simulink model "State_Space_model"  (R2018a)
settings: Solver=ode45  StartTime=0.0  StopTime=5  RelTol=1e-3  EnableMultiTasking=on
values from neighbouring files (symbols this model uses):
  A = [0 0 0   0    0  0     0 ... (first row only)    [State_Space_Pneumatic_Damper.m]
  am1 = 2*zetta*Wn    (= 11.2)    [State_Space_Pneumatic_Damper.m]
  am2 = Wn^2    (= 64)    [State_Space_Pneumatic_Damper.m]
  B = [   c3 ... (first row only)    [State_Space_Pneumatic_Damper.m]
  bm = am2    (= 64)    [State_Space_Pneumatic_Damper.m]
  C = [1 0 0 0 0 0 0 ... (first row only)    [State_Space_Pneumatic_Damper.m]
  D = [0 ... (first row only)    [State_Space_Pneumatic_Damper.m]
  h0 = 150    [State_Space_Pneumatic_Damper.m]
settings Model: Creator=ahmad  LastModifiedBy=Ahmad
settings DataIOCC: LimitDataPoints=on  SaveFormat=Array
settings OptimizationCC: LifeSpan=inf
settings DebuggingCC: UnderspecifiedInitializationDetection=Classic  MergeDetectMultiDrivingBlocksExec=none  SolverPrmCheckMsg=warning  StateNameClashWarn=warning  SFUnexpectedBacktrackingDiag=warning  SFNoUnconditionalDefaultTransitionDiag=warning  SFExecutionAtInitializationDiag=none
settings HardwareCC: ProdBitPerPointer=32  ProdBitPerSizeT=32  ProdBitPerPtrDiffT=32  ProdLargestAtomicFloat=None  ProdIntDivRoundTo=Undefined  ProdEndianess=Unspecified  ProdWordSize=32  ProdHWDeviceType=32-bit Generic
settings ModelReferenceCC: PropagateSignalLabelsOutOfModel=off
settings CodeAppCC: StateflowObjectComments=on
settings GRTTargetCC: TargetLangStandard=C89/C90 (ANSI)  GeneratePreprocessorConditionals=Disable all
settings ConfigComp: CovMetricSettings=dw  CovHtmlReporting=on  CovSaveCumulativeToWorkspaceVar=on  CovSaveSingleToWorkspaceVar=on  CovExternalEMLEnable=off

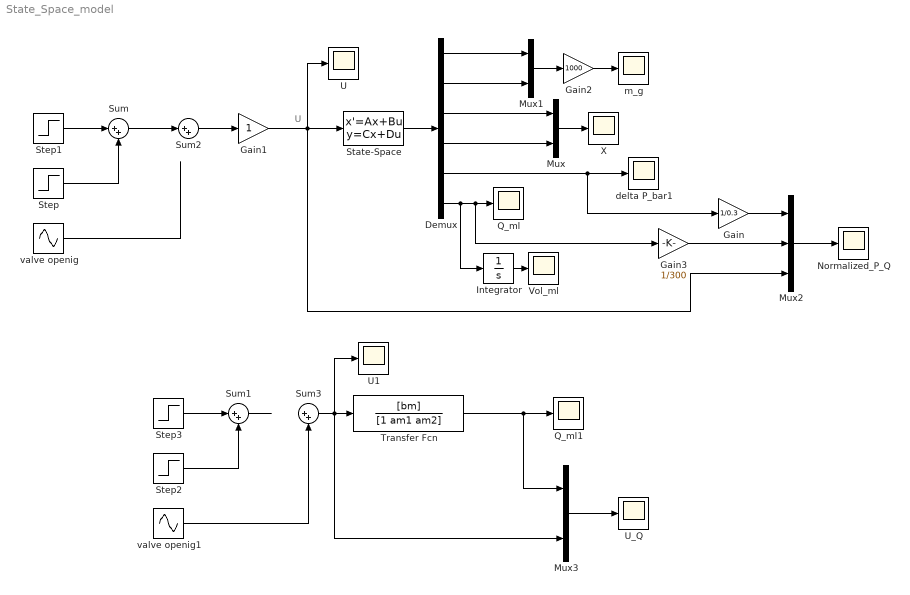
== system State_Space_model ==
  note: U
  Demux : Demux  Outputs=6
  Gain : Gain  Gain=1/0.3
  Gain1 : Gain
  Gain2 : Gain  Gain=1000
  Gain3 : Gain  Gain=1/300
  Integrator : Integrator
  Mux : Mux  Inputs=2
  Mux1 : Mux  Inputs=2
  Mux2 : Mux  Inputs=3
  Mux3 : Mux  Inputs=2
  Normalized_P_Q : Scope
  Q_ml : Scope
  Q_ml1 : Scope
  State-Space : StateSpace  A=A  B=B  C=C  D=D  InitialCondition=[0 0 1.5 1.5 h0/2 h0/2 0]
  Step : Step  Time=0.1  After=-1  SampleTime=0
  Step1 : Step  Time=0  SampleTime=0
  Step2 : Step  Time=0.1  After=-1  SampleTime=0
  Step3 : Step  Time=0  SampleTime=0
  Sum{,1..3} (4 alike) : Sum  Inputs=|++
  Transfer Fcn : TransferFcn  Numerator=[bm]  Denominator=[1 am1 am2]
  U : Scope
  U1 : Scope
  U_Q : Scope
  Vol_ml : Scope
  X : Scope
  delta P_bar1 : Scope
  m_g : Scope
  valve openig : Sin  Phase=pi/2  SampleTime=0
  valve openig1 : Sin  Frequency=8.3  SampleTime=0
  wires:
  State-Space/1 -> Demux/1
  valve openig/1 -> ?
  Demux/6 -> Gain3/1, Q_ml/1, Integrator/1
  Sum/1 -> Sum2/1
  Step/1 -> Sum/2
  Step1/1 -> Sum/1
  Integrator/1 -> Vol_ml/1
  Sum2/1 -> Gain1/1
  Demux/1 -> Mux1/1
  Demux/3 -> Mux/1
  Demux/4 -> Mux/2
  Gain2/1 -> m_g/1
  Demux/2 -> Mux1/2
  Mux/1 -> X/1
  Mux1/1 -> Gain2/1
  Demux/5 -> Gain/1, delta P_bar1/1
  Mux2/1 -> Normalized_P_Q/1
  Gain/1 -> Mux2/1
  Gain3/1 -> Mux2/2
  valve openig1/1 -> Sum3/2
  Sum1/1 -> ?
  Step2/1 -> Sum1/2
  Step3/1 -> Sum1/1
  Sum3/1 -> Mux3/2, U1/1, Transfer Fcn/1
  Transfer Fcn/1 -> Mux3/1, Q_ml1/1
  Mux3/1 -> U_Q/1
  Gain1/1 -> State-Space/1, Mux2/3, U/1
